simulink model "ArduCopter_MinnieLoiterController"  (R2018b)
settings: Solver=FixedStepDiscrete  StartTime=0.0  StopTime=1000  FixedStep=cntrl.sample_time  RelTol=1e-4
libraries: ardupilot_custom_controller_lib x2, axes_transformation_lib x2, fmCopterLoiterIndi_lib x1
settings Model: DataTypeOverride=Single  DataTypeOverrideAppliesTo=Floating-point  Creator=Yannic  LastModifiedBy=yannic
settings SolverCC: ZeroCrossControl=DisableAll
settings DataIOCC: LimitDataPoints=on  SaveOutput=off  SaveTime=off  ReturnWorkspaceOutputs=on
settings OptimizationCC: DefaultParameterBehavior=Inlined  UseFloatMulNetSlope=on  DefaultUnderspecifiedDataType=single  InlineInvariantSignals=on  PassReuseOutputArgsAs=Individual arguments  ZeroExternalMemoryAtStartup=off  ZeroInternalMemoryAtStartup=off  NoFixptDivByZeroProtection=on  EfficientFloat2IntCast=on  LifeSpan=1  OptimizeBlockOrder=speed  DifferentSizesBufferReuse=on
settings DebuggingCC: ReadBeforeWriteMsg=DisableAll  WriteAfterWriteMsg=DisableAll  WriteAfterReadMsg=DisableAll  MultiTaskDSMMsg=none  ParameterTunabilityLossMsg=error  AllowSymbolicDim=off  LibraryContextMissingDiagnostic=none  SFUnexpectedBacktrackingDiag=warning  SFNoUnconditionalDefaultTransitionDiag=warning  SFExecutionAtInitializationDiag=none
settings HardwareCC: ProdBitPerPointer=32  ProdBitPerSizeT=32  ProdBitPerPtrDiffT=32  ProdLargestAtomicInteger=Long  ProdWordSize=32  ProdHWDeviceType=ARM Compatible->ARM 7
settings ModelReferenceCC: UpdateModelReferenceTargets=IfOutOfDate  PropagateSignalLabelsOutOfModel=off
settings SFSimCC: SFSimEcho=off  SimUseLocalCustomCode=off  MATLABDynamicMemAlloc=off
settings RTWCC: SystemTargetFile=ert.tlc  GenCodeOnly=on  TemplateMakefile=ert_default_tmf  GenerateReport=on  RTWUseLocalCustomCode=off  IncludeHyperlinkInReport=on  LaunchReport=on  TargetLang=C++  GenerateTraceInfo=on  GenerateTraceReport=on  GenerateTraceReportSl=on  GenerateTraceReportSf=on  GenerateTraceReportEml=on
settings CodeAppCC: ForceParamTrailComments=on  IgnoreCustomStorageClasses=off  OperatorAnnotations=on  SimulinkDataObjDesc=on  SFDataObjDesc=on  CustomSymbolStrGlobalVar=rt$N$M  CustomSymbolStrType=$N$M  CustomSymbolStrFcn=$N$M$F  CustomSymbolStrMacro=$N$M  InsertBlockDesc=on
settings ERTTargetCC: TargetLangStandard=C++03 (ISO)  GenerateSampleERTMain=on  IncludeMdlTerminateFcn=off  CombineSignalStateStructs=on  SuppressErrorStatus=on  SupportAbsoluteTime=off  MultiInstanceERTCode=on  CodeInterfacePackaging=C++ class  SupportNonFinite=off  SupportComplex=off  SupportVariableSizeSignals=on  ERTHeaderFileRootName=MatlabController$E  ERTSourceFileRootName=MatlabController$E  ERTDataFileRootName=MatlabController_data  InlinedParameterPlacement=NonHierarchical  RootIOFormat=Structure reference  ERTCustomFileTemplate=example_file_process.tlc  ERTFilePackagingFormat=CompactWithDataFile
settings ConfigComp: CovMetricSettings=dw  CovHtmlReporting=on  CovSaveCumulativeToWorkspaceVar=on  CovSaveSingleToWorkspaceVar=on  CovExternalEMLEnable=off

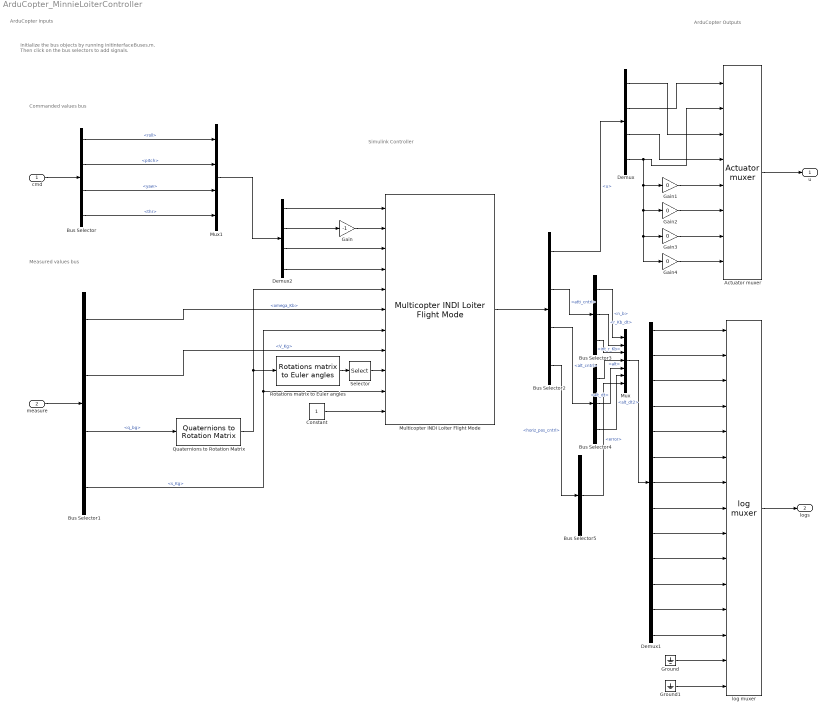
== system ArduCopter_MinnieLoiterController ==
  note: Measured values bus
  note: Initialize the bus objects by running initInterfaceBuses.m.
      | Then click on the bus selectors to add signals.
  note: Commanded values bus
  note: ArduCopter Inputs
  note: ArduCopter Outputs
  note: Simulink Controller
  cmd : Inport  OutDataTypeStr=Bus: cmdBus
  measure : Inport  Port=2  OutDataTypeStr=Bus: measureBus
  Actuator muxer : ardupilot_custom_controller_lib/Actuator muxer
      settings: SourceProductName=LADAC
  Bus Selector : BusSelector  OutputSignals=roll,pitch,yaw,thr
  Bus Selector1 : BusSelector  OutputSignals=omega_Kb,V_Kg,q_bg,s_Kg
  Bus Selector2 : BusSelector  OutputSignals=u,atti_cntrl,alt_cntrl,horiz_pos_cntrl
  Bus Selector3 : BusSelector  OutputSignals=error.n_b,error.r_Kb_dt,error.int_r_Kb
  Bus Selector4 : BusSelector  OutputSignals=error.alt,error.alt_dt,error.alt_dt2
  Bus Selector5 : BusSelector  OutputSignals=error
  Constant : Constant
  Demux : Demux
  Demux1 : Demux  Outputs=13
  Demux2 : Demux
  Gain : Gain  Gain=-1
  Gain{1..4} (4 alike) : Gain  Gain=0
  Ground : Ground
  Ground1 : Ground
  Multicopter INDI Loiter Flight Mode : fmCopterLoiterIndi_lib/Multicopter INDI Loiter Flight Mode  fm=fm_loiter
      settings: SourceProductName=LADAC
  Mux : Mux  Inputs=7
  Mux1 : Mux
  Quaternions to Rotation Matrix : axes_transformation_lib/Quaternions to Rotation Matrix  SystemSampleTime=-1
      settings: SourceProductName=LADAC
  Rotations matrix to Euler angles : axes_transformation_lib/Rotations matrix to Euler angles  SystemSampleTime=-1
      settings: SourceProductName=LADAC
  Selector : Selector  InputPortWidth=3  IndexOptions=Index vector (dialog)  Indices=3  OutputSizes=1
  log muxer : ardupilot_custom_controller_lib/log muxer
      settings: SourceProductName=LADAC
  u : Outport
  logs : Outport  Port=2
  wires:
  cmd/1 -> Bus Selector/1
  measure/1 -> Bus Selector1/1
  Bus Selector/1 -> Mux1/1  "<roll>"
  Bus Selector/2 -> Mux1/2  "<pitch>"
  Bus Selector/3 -> Mux1/3  "<yaw>"
  Bus Selector/4 -> Mux1/4  "<thr>"
  Actuator muxer/1 -> u/1
  log muxer/1 -> logs/1
  Demux/4 -> Actuator muxer/2, Gain1/1, Gain4/1, Gain3/1, Gain2/1
  Gain1/1 -> Actuator muxer/5
  Demux/3 -> Actuator muxer/4
  Demux/2 -> Actuator muxer/1
  Demux1/1 -> log muxer/1
  Demux1/2 -> log muxer/2
  Demux1/3 -> log muxer/3
  Demux1/4 -> log muxer/4
  Demux1/5 -> log muxer/5
  Demux1/6 -> log muxer/6
  Demux1/7 -> log muxer/7
  Demux1/8 -> log muxer/8
  Demux1/9 -> log muxer/9
  Demux1/10 -> log muxer/10
  Demux1/11 -> log muxer/11
  Demux1/12 -> log muxer/12
  Demux1/13 -> log muxer/13
  Ground/1 -> log muxer/14
  Ground1/1 -> log muxer/15
  Gain/1 -> Multicopter INDI Loiter Flight Mode/2
  Quaternions to Rotation Matrix/1 -> Multicopter INDI Loiter Flight Mode/5, Rotations matrix to Euler angles/1
  Bus Selector1/2 -> Multicopter INDI Loiter Flight Mode/8  "<V_Kg>"
  Demux2/4 -> Multicopter INDI Loiter Flight Mode/4
  Rotations matrix to Euler angles/1 -> Selector/1
  Mux1/1 -> Demux2/1
  Bus Selector1/1 -> Multicopter INDI Loiter Flight Mode/6  "<omega_Kb>"
  Demux2/2 -> Gain/1
  Demux2/3 -> Multicopter INDI Loiter Flight Mode/3
  Bus Selector1/4 -> Multicopter INDI Loiter Flight Mode/10, Multicopter INDI Loiter Flight Mode/7  "<s_Kg>"
  Constant/1 -> Multicopter INDI Loiter Flight Mode/11
  Demux2/1 -> Multicopter INDI Loiter Flight Mode/1
  Bus Selector1/3 -> Quaternions to Rotation Matrix/1  "<q_bg>"
  Multicopter INDI Loiter Flight Mode/1 -> Bus Selector2/1
  Bus Selector2/1 -> Demux/1  "<u>"
  Gain2/1 -> Actuator muxer/6
  Gain3/1 -> Actuator muxer/7
  Gain4/1 -> Actuator muxer/8
  Demux/1 -> Actuator muxer/3
  Bus Selector2/2 -> Bus Selector3/1  "<atti_cntrl>"
  Bus Selector2/3 -> Bus Selector4/1  "<alt_cntrl>"
  Bus Selector2/4 -> Bus Selector5/1  "<horiz_pos_cntrl>"
  Bus Selector5/1 -> Mux/7  "<error>"
  Bus Selector3/1 -> Mux/1  "<n_b>"
  Bus Selector3/3 -> Mux/3  "<int_r_Kb>"
  Bus Selector4/1 -> Mux/4  "<alt>"
  Bus Selector4/3 -> Mux/6  "<alt_dt2>"
  Mux/1 -> Demux1/1
  Bus Selector4/2 -> Mux/5  "<alt_dt>"
  Bus Selector3/2 -> Mux/2  "<r_Kb_dt>"
  Selector/1 -> Multicopter INDI Loiter Flight Mode/9
